simulink library "mcl"  (R2020b)
settings: Solver=VariableStepAuto  StartTime=0.0  StopTime=10.0  RelTol=1e-3
settings Model: Creator=sai  LastModifiedBy=sai

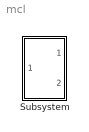
== system mcl ==
  Subsystem : Subsystem  mask{A=33, B=44}
      mask Display: image('download.jpg'); % Use "Edit Image" on toolstrip to change.

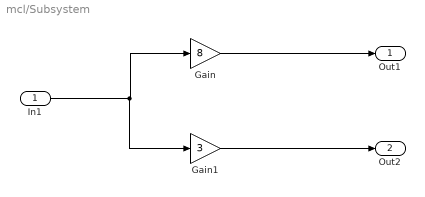
== system mcl/Subsystem ==
  In1 : Inport
  Gain : Gain  Gain=8
  Gain1 : Gain  Gain=3
  Out1 : Outport
  Out2 : Outport  Port=2
  wires:
  In1/1 -> Gain1/1, Gain/1
  Gain1/1 -> Out2/1
  Gain/1 -> Out1/1
